simulink model "timestwo_sim"  (Simulink 7.6)
settings: Solver=FixedStepDiscrete  StartTime=0.0  StopTime=ps_simEndTime  FixedStep=ps_simStepTime  RelTol=1e-3
settings Model: Creator=CNFELUO1  LastModifiedBy=CNFELUO1

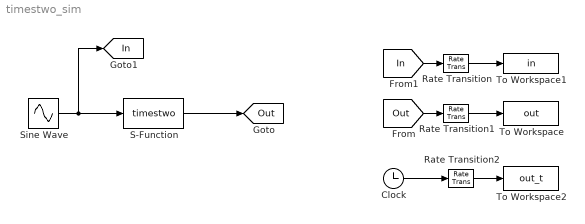
== system timestwo_sim ==
  Clock : Clock
      settings: Decimation=10
  Rate Transition : RateTransition  OutPortSampleTime=ps_measSamplingTime
  Rate Transition1 : RateTransition  OutPortSampleTime=ps_measSamplingTime
  Rate Transition2 : RateTransition  OutPortSampleTime=ps_measSamplingTime
  S-Function : S-Function  FunctionName=timestwo  EnableBusSupport=off
  Sine Wave : Sin  Frequency=50*2*3.14  SampleTime=0
  To Workspace : ToWorkspace  VariableName=out  SampleTime=-1  SaveFormat=Array
  To Workspace1 : ToWorkspace  VariableName=in  SampleTime=-1  SaveFormat=Array
  To Workspace2 : ToWorkspace  VariableName=out_t  SampleTime=-1  SaveFormat=Array
  tag scope: In=global, Out=global
  wires:
  Sine Wave/1 -> S-Function/1, [In]
  S-Function/1 -> [Out]
  [In] -> Rate Transition/1
  Rate Transition/1 -> To Workspace1/1
  [Out] -> Rate Transition1/1
  Rate Transition1/1 -> To Workspace/1
  Clock/1 -> Rate Transition2/1
  Rate Transition2/1 -> To Workspace2/1
